simulink model "SRLatchWithNOR"  (R2024b)
settings: Solver=VariableStepAuto  StartTime=0.0  StopTime=inf  RelTol=1e-3
settings Model: Creator=Soochan Kim  LastModifiedBy=Soochan Kim

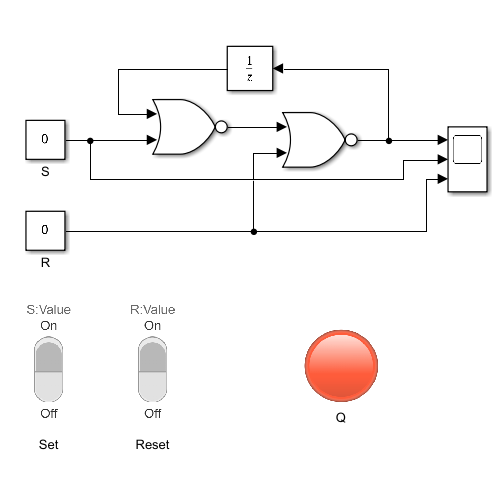
[thumbnail: Simulink's stored preview of the top-level diagram]
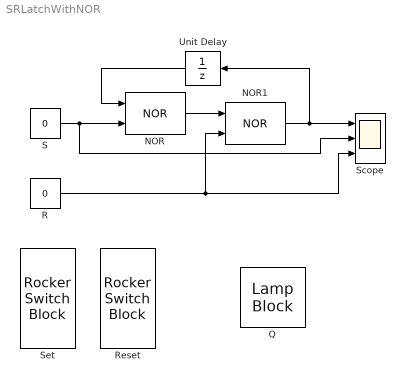
== system SRLatchWithNOR ==
  NOR : Logic  Operator=NOR  IconShape=distinctive  AllPortsSameDT=off  OutDataTypeStr=boolean
  NOR1 : Logic  Operator=NOR  IconShape=distinctive  AllPortsSameDT=off  OutDataTypeStr=boolean
  Q : LampBlock  LabelPosition=Hide
  R : Constant  Value=0
  Reset : RockerSwitchBlock
      settings: Values={{'Off', 'On'}, [0 1]}
  S : Constant  Value=0
  Scope : Scope  NumInputPorts=3
  Set : RockerSwitchBlock
      settings: Values={{'Off', 'On'}, [0 1]}
  Unit Delay : UnitDelay  SampleTime=-1  HasFrameUpgradeWarning=on
  wires:
  NOR/1 -> NOR1/1
  NOR1/1 -> Unit Delay/1, Scope/1
  S/1 -> Scope/2, NOR/2
  R/1 -> Scope/3, NOR1/2
  Unit Delay/1 -> NOR/1
